simulink model "gps_tracking_costas_cic_hwcosim"  (R2018a)
settings: Solver=VariableStepAuto  StartTime=0.0  StopTime=8*8e4/16367600  RelTol=1e-3
undefined symbols (not defined in the file): A, N
libraries: xbsIndex_r4 x4, dspsrcs4 x1, JTAGRuntimeCosim_r4 x1
settings Model: Creator=Doc_v  LastModifiedBy=Doc_v

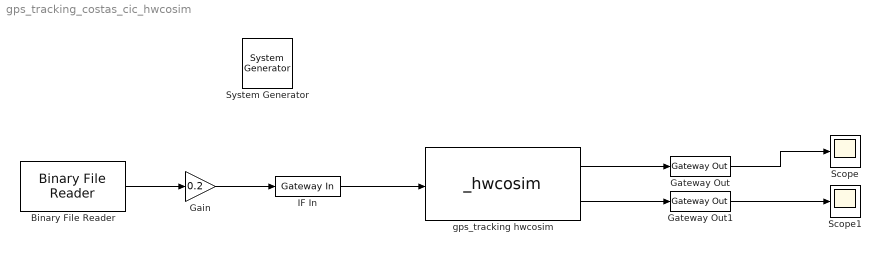
== system gps_tracking_costas_cic_hwcosim ==
  " System Generator" : xbsIndex_r4/ System Generator  Tag=genX  xilinxfamily=kintex7  part=xc7k325t  speed=-2  package=ffg900  synthesis_tool=Vivado  clock_wrapper=Clock Enables  directory=./gps_tracking  proj_type=Vivado  Synth_file=Vivado Synthesis Defaults  Impl_file=Vivado Implementation Defaults  testbench=off  simulink_period=1/16367600  sysclk_period=10  dcm_input_clock_period=10  incr_netlist=off  trim_vbits=Everywhere in SubSystem  dbl_ovrd=According to Block Masks  core_generation=According to Block Masks  run_coregen=off  deprecated_control=off  eval_field=0  block_type=sysgen
  Binary File Reader : dspsrcs4/Binary File Reader  Filename=D:\QQfile\myGNSS_NO_PN.bin  HeaderStructure=struct([])  DataType=int8  SamplesPerFrame=1  IsDataComplex=off  NumChannels=1  OutputEOF=off  SampleTime=1/16367600  SimulateUsing=Code generation
      settings: SourceProductName=DSP System Toolbox  SourceProductBaseCode=DS
  Gain : Gain  Gain=0.2
  Gateway Out : xbsIndex_r4/Gateway Out  inherit_from_input=off  hdl_port=on  rows=1  columns=1  UseAsDAC=off  DACChannel='1'  interface=None  automatic_assignment=on  address_offset=hex2dec('00')  intf_name=''  intf_description=''  timing_constraint=None  locs_specified=off  LOCs={}  io_standard={}  block_type=gatewayout
  Gateway Out1 : xbsIndex_r4/Gateway Out  inherit_from_input=off  hdl_port=on  rows=1  columns=1  UseAsDAC=off  DACChannel='1'  interface=None  automatic_assignment=on  address_offset=hex2dec('00')  intf_name=''  intf_description=''  timing_constraint=None  locs_specified=off  LOCs={}  io_standard={}  block_type=gatewayout
  IF In : xbsIndex_r4/Gateway In  gui_display_data_type=Fixed-point  arith_type="Signed  (2's comp)"  n_bits=16  bin_pt=15  preci_type=Single  exp_width=8  frac_width=24  rows=1  columns=1  quantization="Round  (unbiased: +/- Inf)"  overflow=Flag as error  period=1/16367600  UseAsADC=off  ADCChannel='1'  interface=None  automatic_assignment=on  address_offset=hex2dec('00')  intf_name=''  intf_description=''  default_value=0  timing_constraint=None  locs_specified=off  LOCs={}  io_standard={}  inherit_from_input=off  hdl_port=on  dbl_ovrd=off  block_type=gatewayin
  Scope : Scope
  Scope1 : Scope
  gps_tracking hwcosim : JTAGRuntimeCosim_r4/_hwcosim  clkSrc=Single Stepped  hasCombinationalPath=on  bitfileName=E:/sysgen_workspace/gps_tracking_costas_cic_hwcosim/gps_tracking.bit  skipConfig=off  dispPartInfo=on  useZynqReconfigScript=on  cable=Auto Detect  speed=N/A  cablePort=N/A  cableLocation=Local  shareCable=off  design_xtable=|  engineDll=JTAGCosimEngine.dll  cableWaitTime=10  bscanPos=-1  IRLengths=[]  useWaitBox=1  hasBufgmux=on  Scheme=Cosim  useCmdProc=1  hasProc=0  useImpact=0  printLogFile=0  userChain=2  block_type=jtagcosim
      | {
      |     'clkWrapper' => 'gps_tracking',
      |     'burstMode' => false,
      |     'burstFifoDepth' => '1024',
      |     'shared_memories' => {},
      |     'clocksGcd' => 1,
      |     'device' => {
      |       'family' => 'kintex7',
      |       'part' => 'xc7k325t',
      |       'package' => 'ffg900',
      |       'speed' => '-2',
      |     },
      |     'ports' => {
      |       'if_in' => {
      |         'direction' => 'in',
      |         'width' => 16,
      |         'name' => 'if_in',
      |         'period' => 1,
      |         'icon_text' => 'IF In',
      |         'type' => 'Fix_16_15',
      |         'arithmetic_type' => 'xlSigned',
      |         'dat_file' => 'gps_tracking_if_in.dat',
      |         'bin_pt' => 15,
      |         'addr_offset' => 0,
      |         'bd_port_index' => 0,
      |       },
      |       'gateway_out1' => {
      |         'direction' => 'out',
      |         'width' => 16,
      |         'name' => 'gateway_out1',
      |         'period' => 1,
      |         'icon_text' => 'Gateway Out1',
      |         'type' => 'Fix_16_15',
      |         'arithmetic_type' => 'xlSigned',
      |         'dat_file' => 'gps_tracking_gateway_out1.dat',
      |         'bin_pt' => 15,
      |         'addr_offset' => 4,
      |         'bd_port_index' => 0,
      |       },
      |       'gateway_out5' => {
      |         'direction' => 'out',
      |         'width' => 32,
      |         'name' => 'gateway_out5',
      |         'period' => 1,
      |         'icon_text' => 'Gateway Out5',
      |         'type' => 'Fix_32_15',
      |         'arithmetic_type' => 'xlSigned',
      |         'dat_file' => 'gps_tracking_gateway_out5.dat',
      |         'bin_pt' => 15,
      |         'addr_offset' => 8,
      |         'bd_port_index' => 1,
      |       },
      |     },
      |   }
  wires:
  IF In/1 -> gps_tracking hwcosim/1
  gps_tracking hwcosim/1 -> Gateway Out/1
  Gateway Out/1 -> Scope/1
  Gateway Out1/1 -> Scope1/1
  gps_tracking hwcosim/2 -> Gateway Out1/1
  Binary File Reader/1 -> Gain/1
  Gain/1 -> IF In/1
